simulink model "plant"  (R2023b)
settings: Solver=VariableStepAuto  StartTime=0.0  StopTime=100  RelTol=1e-3
values from neighbouring files (symbols this model uses):
  A = [ ... (first row only)    [controller_mass_damper.m]    (also in main.m; mass_damper_controllable.m; mass_damper_observable.m; observer_mass_damper.m)
  alpha = 0.5    [main.m]
  B = [0; 1/m; 0; 0]    [controller_mass_damper.m]    (also in main.m = [0; -1/L; 0; 1]; mass_damper_controllable.m; mass_damper_observable.m; observer_mass_damper.m)
  C = [1, 0, 0, 0]    [controller_mass_damper.m]    (also in main.m = [; mass_damper_controllable.m; mass_damper_observable.m; observer_mass_damper.m)
  D = 0    [controller_mass_damper.m]    (also in main.m = [; mass_damper_controllable.m; mass_damper_observable.m; observer_mass_damper.m)
  g = 9.8    [main.m]    (also in sim_invpendulum.m)
  K = place(A, B, p)    [controller_mass_damper.m]    (also in main.m = place(A, B, conPoles); mass_damper_controllable.m = 9; mass_damper_observable.m = 9; observer_mass_damper.m = 9)
  Ki = 15*r_con_p    [main.m]    (also in sim_invpendulum.m = Ktot(1))
  L = 0.5    [main.m]    (also in observer_mass_damper.m = L'; sim_invpendulum.m)
  Lo = place(A', C', obsPoles)'    [main.m]    (also in sim_invpendulum.m)
settings Model: Creator=kaitlin  LastModifiedBy=kaitlin

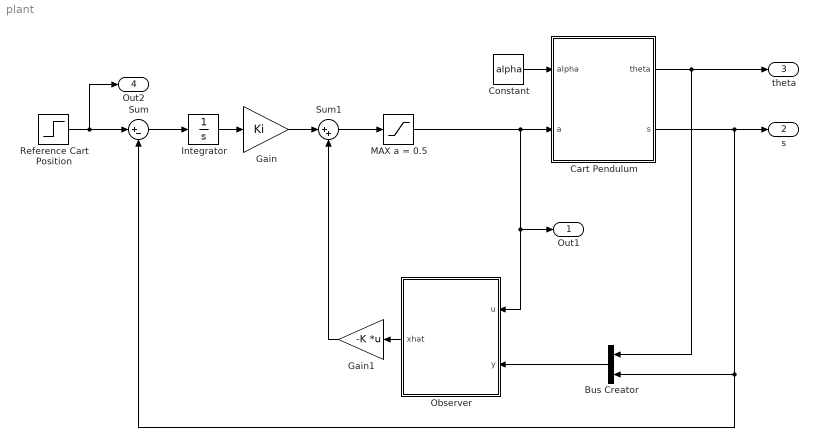
== system plant ==
  Bus Creator : BusCreator  Inputs=2
  Cart Pendulum : Subsystem
  Constant : Constant  Value=alpha
  Gain : Gain  Gain=Ki
  Gain1 : Gain  Gain=-K  Multiplication=Matrix(K*u)
  Integrator : Integrator
  MAX a = 0.5 : Saturate
  Observer : Subsystem
  Reference Cart Position : Step  SampleTime=0
  Sum : Sum  Inputs=|+-
  Sum1 : Sum  Inputs=|++
  Out1 : Outport  SignalName=a(t)
  s : Outport  Port=2  SignalName=s(t)
  theta : Outport  Port=3  SignalName=theta(t)
  Out2 : Outport  Port=4  SignalName=r(t)
  wires:
  Reference Cart Position/1 -> Out2/1, Sum/1
  Gain/1 -> Sum1/1
  Integrator/1 -> Gain/1
  Sum/1 -> Integrator/1
  Gain1/1 -> Sum1/2
  Sum1/1 -> MAX a = 0.5/1
  MAX a = 0.5/1 -> Observer/1(u), Out1/1, Cart Pendulum/2(a)
  Cart Pendulum/2(s) -> Sum/2, Bus Creator/2, s/1
  Cart Pendulum/1(theta) -> Bus Creator/1, theta/1
  Observer/1(xhat) -> Gain1/1
  Bus Creator/1 -> Observer/2(y)
  Constant/1 -> Cart Pendulum/1(alpha)

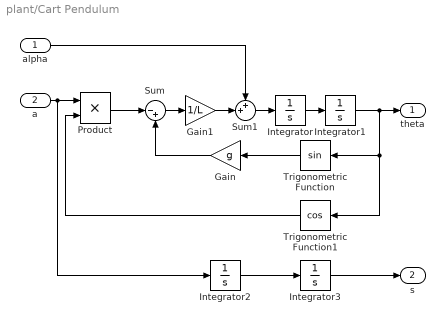
== system plant/Cart Pendulum ==
  alpha : Inport
  a : Inport  Port=2
  Gain : Gain  Gain=g
  Gain1 : Gain  Gain=1/L
  Integrator{,1..3} (4 alike) : Integrator
  Product : Product
  Sum : Sum  Inputs=|-+
  Sum1 : Sum  Inputs=++|
  Trigonometric Function : Trigonometry
  Trigonometric Function1 : Trigonometry  Operator=cos
  theta : Outport
  s : Outport  Port=2
  wires:
  Product/1 -> Sum/1
  Trigonometric Function/1 -> Gain/1
  Gain/1 -> Sum/2
  alpha/1 -> Sum1/1
  Trigonometric Function1/1 -> Product/2
  Integrator/1 -> Integrator1/1
  Sum1/1 -> Integrator/1
  Integrator1/1 -> theta/1, Trigonometric Function1/1, Trigonometric Function/1
  Integrator2/1 -> Integrator3/1
  a/1 -> Product/1, Integrator2/1
  Integrator3/1 -> s/1
  Sum/1 -> Gain1/1
  Gain1/1 -> Sum1/2

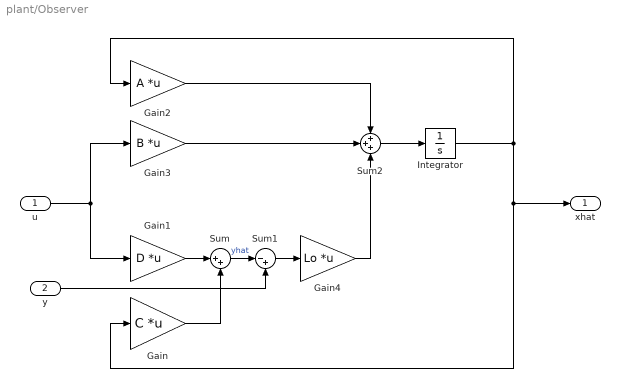
== system plant/Observer ==
  u : Inport
  y : Inport  Port=2
  Gain : Gain  Gain=C  Multiplication=Matrix(K*u)
  Gain1 : Gain  Gain=D  Multiplication=Matrix(K*u)
  Gain2 : Gain  Gain=A  Multiplication=Matrix(K*u)
  Gain3 : Gain  Gain=B  Multiplication=Matrix(K*u)
  Gain4 : Gain  Gain=Lo  Multiplication=Matrix(K*u)
  Integrator : Integrator
  Sum : Sum  Inputs=|++
  Sum1 : Sum  Inputs=|-+
  Sum2 : Sum  Inputs=+++
  xhat : Outport
  wires:
  Gain/1 -> Sum/2
  Gain1/1 -> Sum/1
  Sum/1 -> Sum1/1  "yhat"
  u/1 -> Gain3/1, Gain1/1
  Gain2/1 -> Sum2/1
  Gain3/1 -> Sum2/2
  y/1 -> Sum1/2
  Sum1/1 -> Gain4/1
  Sum2/1 -> Integrator/1
  Integrator/1 -> Gain/1, xhat/1, Gain2/1
  Gain4/1 -> Sum2/3
